simulink model "SimForces2022a"  (R2022a)
settings: Solver=daessc  StartTime=0.0  StopTime=10  FixedStep=0.001  RelTol=1e-4
values from neighbouring files (symbols this model uses):
  Bc1_V = [0;0;0;0;0;0]    [initializeSimulationGP.m]
  D22F = [0;0;0;0;0;0]    [initializeSimulationGP.m]
  filtDV = init2ndOrderLowPassFilter(35*2*pi,1,controller.dT)    [initializeLowPassFilters.m]
  filtEnc = init2ndOrderLowPassFilter(35*2*pi,1,controller.dT)    [initializeLowPassFilters.m]
undefined symbols (not defined in the file or in its folder): aux, B11_r_B11Tc1, B11_V, B11Ftot, B12_r_B12Tc2, B12_Rot_Tc2, B12_U_Tc2, B12_V, B12Ftot, B31_r_B31B41, B31_V, B31FTot, B32_r_B32B42, B32_Rot_B42, B32_U_B42, B32_V, B32FTot, B41_r_B41Tc1, B41_V, B41FTot, B42_r_B42Tc2, B42_Rot_Tc2, B42_U_Tc2, B42_V, B42FTot, B52_r_B52P32, B52_Rot_P32, B52_U_P32, B52_V, B52Ftot, Bc1_r_Bc1B11, Bc1_r_Bc1B31, Bc1FTot, Bc2_r_Bc2B12, Bc2_r_Bc2B32, Bc2_Rot_B12, Bc2_Rot_B32, Bc2_U_B12, Bc2_U_B32, Bc2_V, Bc2Tot, controller, cyl1, cyl2, D22_V, dq1, dq11, dq12, dq2, dq21, dq22, dx1, dx2, dxt2, fc1, fc1r, fc2, fc2r, fct2, fct2r ... (+61)
libraries: sm_lib x32, nesl_utility x20
(part 7 of 7)

== matlab function SimForces2022a/sbVDCController/sbFormAnalyticQuantities/sbRevoluteSegment1/sbGeomPropRS1/sbLiftPistonVelocity/liftPistonVelocity ==
  data: dq1 input; x1 input; q1 input; dx1 output; geom parameter; cyl1 parameter
function dx1 = liftPistonVelocity(dq1, x1, q1, geom, cyl1)

    % Calculates lift piston velocity per the paper equation (21).
    dx1 = -(geom.L1*geom.L11*sin(q1))/(x1+cyl1.x0)*dq1;

end

== matlab function SimForces2022a/sbVDCController/sbFormAnalyticQuantities/sbRevoluteSegment1/sbGeomPropRS1/sbq11AngleVelocity/q11AngleRate ==
  data: x1 input; q11 input; dx1 input; dq11 output; geom parameter; cyl1 parameter
function dq11 = q11AngleRate(x1, q11, dx1, geom, cyl1)
    
    % Calculates q11 angle rate per the paper equation (22).
    dq11 = -((x1+cyl1.x0)-geom.L1*cos(q11))/((x1+cyl1.x0)*geom.L1*sin(q11))*dx1;

end

== matlab function SimForces2022a/sbVDCController/sbFormAnalyticQuantities/sbRevoluteSegment1/sbGeomPropRS1/sbq12AngleRate/q12AngleRate ==
  data: x1 input; q12 input; dx1 input; dq12 output; geom parameter; cyl1 parameter
function dq12 = q12AngleRate(x1, q12, dx1, geom, cyl1)

    % Calculates q12 angle rate per the paper equation (23). 
    dq12 = -((x1+cyl1.x0)-geom.L11*cos(q12))/((x1+cyl1.x0)*geom.L11*sin(q12))*dx1;

end

== matlab function SimForces2022a/sbVDCController/sbFormAnalyticQuantities/sbRevoluteSegment1/sbPosVecsRS1/B31_r_B31B41 ==
  data: x1 input; B31_r_B31B41 output; posVec parameter
function B31_r_B31B41 = B31_r_B31B41(x1, posVec)

    % position vector of {B41} frame at lift piston tip w.r.t. {B31} frame at 
    % lift cylinder connection point [m]
    B31_r_B31B41 = posVec.B31_r_B31B31p + [x1;0;0];

end

== matlab function SimForces2022a/sbVDCController/sbFormAnalyticQuantities/sbRevoluteSegment1/sbGeomPropRS1/sbLiftPistonStroke/liftPistonStroke ==
  data: q1 input; x1 output; geom parameter; cyl1 parameter
function x1 = liftPistonStroke(q1, geom, cyl1)

    % Calculates lift piston stroke per the paper equation (18).
    x1 = sqrt(geom.L1*geom.L1+geom.L11*geom.L11+2*geom.L1*geom.L11*cos(q1))-cyl1.x0;

end

== matlab function SimForces2022a/sbVDCController/sbFormAnalyticQuantities/sbRevoluteSegment1/sbRotMatsRS1/B41_Rot_Tc1 ==
  data: q12 input; B41_Rot_Tc1 output
function B41_Rot_Tc1 = B41_Rot_Tc1(q12)

B41_Rot_Tc1 = [+cos(q12) -sin(q12) 0;...
               +sin(q12) +cos(q12) 0;...
                   0        0      1];

== matlab function SimForces2022a/sbVDCController/sbFormAnalyticQuantities/sbRevoluteSegment1/sbRotMatsRS1/Bc1_Rot_B11 ==
  data: q1 input; Bc1_Rot_B11 output
function Bc1_Rot_B11 = Bc1_Rot_B11(q1)

Bc1_Rot_B11 = [+cos(q1) -sin(q1) 0;...
               +sin(q1) +cos(q1) 0;...
                  0        0     1];

== matlab function SimForces2022a/sbVDCController/sbFormAnalyticQuantities/sbRevoluteSegment1/sbRotMatsRS1/Bc1_Rot_B31 ==
  data: q11 input; Bc1_Rot_B31 output
function Bc1_Rot_B31 = Bc1_Rot_B31(q11)

Bc1_Rot_B31 = [+cos(q11) -sin(q11) 0;...
               +sin(q11) +cos(q11) 0;...
                   0         0     1];

== matlab function SimForces2022a/sbVDCController/sbFormAnalyticQuantities/sbRevoluteSegment1/sbUMatsRS1/B11_U_Tc1 ==
  data: B11_r_B11Tc1 input; B11_U_Tc1 output; B11_Rot_Tc1 input
function B11_U_Tc1 = B11_U_Tc1(B11_r_B11Tc1, B11_Rot_Tc1)

B11_U_Tc1 = [B11_Rot_Tc1,                    zeros(3);...
             dual(B11_r_B11Tc1)*B11_Rot_Tc1, B11_Rot_Tc1];
   
end
   
function dual_r = dual(ArAB)

dual_r = [0,  -ArAB(3), ArAB(2);...
          ArAB(3), 0, -ArAB(1);...
          -ArAB(2), ArAB(1), 0];

end

== matlab function SimForces2022a/sbVDCController/sbFormAnalyticQuantities/sbRevoluteSegment1/sbUMatsRS1/B31_U_B41 ==
  data: B31_r_B31B41 input; B31_U_B41 output; B31_Rot_B41 input
function B31_U_B41 = B31_U_B41(B31_r_B31B41, B31_Rot_B41)

B31_U_B41 = [B31_Rot_B41,                    zeros(3);...
             dual(B31_r_B31B41)*B31_Rot_B41, B31_Rot_B41];
   
end
   
function dual_r = dual(ArAB)

dual_r = [0,  -ArAB(3), ArAB(2);...
          ArAB(3), 0, -ArAB(1);...
          -ArAB(2), ArAB(1), 0];

end

== matlab function SimForces2022a/sbVDCController/sbFormAnalyticQuantities/sbRevoluteSegment1/sbUMatsRS1/B41_U_Tc1 ==
  data: B41_r_B41Tc1 input; B41_U_Tc1 output; B41_Rot_Tc1 input
function B41_U_Tc1 = B41_U_Tc1(B41_r_B41Tc1, B41_Rot_Tc1)

B41_U_Tc1 = [B41_Rot_Tc1,                    zeros(3);...
             dual(B41_r_B41Tc1)*B41_Rot_Tc1, B41_Rot_Tc1];
   
end
   
function dual_r = dual(ArAB)

dual_r = [0,  -ArAB(3), ArAB(2);...
          ArAB(3), 0, -ArAB(1);...
          -ArAB(2), ArAB(1), 0];

end

== matlab function SimForces2022a/sbVDCController/sbFormAnalyticQuantities/sbRevoluteSegment1/sbUMatsRS1/Bc1_U_B11 ==
  data: Bc1_r_Bc1B11 input; Bc1_U_B11 output; Bc1_Rot_B11 input
function Bc1_U_B11 = Bc1_U_B11(Bc1_r_Bc1B11, Bc1_Rot_B11)

Bc1_U_B11 = [Bc1_Rot_B11,                    zeros(3);...
             dual(Bc1_r_Bc1B11)*Bc1_Rot_B11, Bc1_Rot_B11];
   
end
   
function dual_r = dual(ArAB)

dual_r = [0,  -ArAB(3), ArAB(2);...
          ArAB(3), 0, -ArAB(1);...
          -ArAB(2), ArAB(1), 0];

end

== matlab function SimForces2022a/sbVDCController/sbFormAnalyticQuantities/sbRevoluteSegment1/sbUMatsRS1/Bc1_U_B31 ==
  data: Bc1_r_Bc1B31 input; Bc1_U_B31 output; Bc1_Rot_B31 input
function Bc1_U_B31 = Bc1_U_B31(Bc1_r_Bc1B31, Bc1_Rot_B31)

Bc1_U_B31 = [Bc1_Rot_B31,                    zeros(3);...
             dual(Bc1_r_Bc1B31)*Bc1_Rot_B31, Bc1_Rot_B31];
   
end
   
function dual_r = dual(ArAB)

dual_r = [0,  -ArAB(3), ArAB(2);...
          ArAB(3), 0, -ArAB(1);...
          -ArAB(2), ArAB(1), 0];

end

== matlab function SimForces2022a/sbVDCController/sbFormAnalyticQuantities/sbRevoluteSegment1/sbUMatsRS1/Tc1_U_Bc2 ==
  data: Tc1_r_Tc1Bc2 input; Tc1_U_Bc2 output; Tc1_Rot_Bc2 input
function Tc1_U_Bc2 = Tc1_U_Bc2(Tc1_r_Tc1Bc2, Tc1_Rot_Bc2)

Tc1_U_Bc2 = [Tc1_Rot_Bc2,                    zeros(3);...
             dual(Tc1_r_Tc1Bc2)*Tc1_Rot_Bc2, Tc1_Rot_Bc2];
   
end
   
function dual_r = dual(ArAB)

dual_r = [0,  -ArAB(3), ArAB(2);...
          ArAB(3), 0, -ArAB(1);...
          -ArAB(2), ArAB(1), 0];

end

== matlab function SimForces2022a/sbVDCController/sbFormAnalyticQuantities/sbPrismaticSegment2/sbPosVecsPS2/P22_r_P22B52 ==
  data: xt2 input; P22_r_P22B52 output; posVec parameter
function P22_r_P22B52 = P22_r_P22B52(xt2, posVec)

    % position vector of {B41} frame at lift piston tip w.r.t. {B31} frame at 
    % lift cylinder connection point [m]
    P22_r_P22B52 = posVec.P22_r_P22P22p + [xt2; 0; 0];

end

== matlab function SimForces2022a/sbVDCController/sbFormAnalyticQuantities/sbPrismaticSegment2/sbUMatsPS2/B52_U_P32 ==
  data: B52_r_B52B32 input; B52_U_P32 output; B52_Rot_B32 input
function B52_U_P32 = B52_U_P32(B52_r_B52B32, B52_Rot_B32)

B52_U_P32 = [B52_Rot_B32,                    zeros(3);...
             dual(B52_r_B52B32)*B52_Rot_B32, B52_Rot_B32];
   
end
   
function dual_r = dual(ArAB)

dual_r = [0,  -ArAB(3), ArAB(2);...
          ArAB(3), 0, -ArAB(1);...
          -ArAB(2), ArAB(1), 0];

end

== matlab function SimForces2022a/sbVDCController/sbFormAnalyticQuantities/sbPrismaticSegment2/sbUMatsPS2/P22_U_B52 ==
  data: P22_r_P22B52 input; P22_U_B52 output; P22_Rot_B52 input
function P22_U_B52 = P22_U_B52(P22_r_P22B52, P22_Rot_B52)

P22_U_B52 = [P22_Rot_B52,                    zeros(3);...
             dual(P22_r_P22B52)*P22_Rot_B52, P22_Rot_B52];
   
end
   
function dual_r = dual(ArAB)

dual_r = [0,  -ArAB(3), ArAB(2);...
          ArAB(3), 0, -ArAB(1);...
          -ArAB(2), ArAB(1), 0];

end

== matlab function SimForces2022a/sbVDCController/sbFormAnalyticQuantities/sbRevoluteSegment1/sbGeomPropRS1/sbq11AngleValue/q11AngleValue ==
  data: x1 input; q11 output; geom parameter; cyl1 parameter
function q11 = q11AngleValue(x1, geom, cyl1)

    % Calculates q11-angle per the paper equation (19).
    q11 = -acos((geom.L11*geom.L11-(x1+cyl1.x0)*(x1+cyl1.x0)-geom.L1*geom.L1)/(-2*(x1+cyl1.x0)*geom.L1));

end

== matlab function SimForces2022a/sbVDCController/sbFormAnalyticQuantities/sbPrismaticSegment2/sbUMatsPS2/P32_U_D22 ==
  data: P32_r_P32D22 input; P32_U_D22 output; P32_Rot_D22 input
function P32_U_D22 = P32_U_D22(P32_r_P32D22, P32_Rot_D22)

P32_U_D22 = [P32_Rot_D22,                    zeros(3);...
              dual(P32_r_P32D22)*P32_Rot_D22, P32_Rot_D22];
   
end
   
function dual_r = dual(ArAB)

dual_r = [0,  -ArAB(3), ArAB(2);...
          ArAB(3), 0, -ArAB(1);...
          -ArAB(2), ArAB(1), 0];

end

== matlab function SimForces2022a/sbVDCController/sbFormAnalyticQuantities/sbRevoluteSegment2/sbPosVecsRS2/B32_r_B32B42 ==
  data: x2 input; B32_r_B32B42 output; posVec parameter
function B32_r_B32B42 = B32_r_B32B42(x2, posVec)

B32_r_B32B42 = posVec.B32_r_B32B32p + [x2;0;0];

== matlab function SimForces2022a/sbVDCController/sbFormAnalyticQuantities/sbRevoluteSegment2/sbRotMatsRS2/B42_Rot_Tc2 ==
  data: q22 input; B42_Rot_Tc2 output
function B42_Rot_Tc2 = B42_Rot_Tc2(q22)

B42_Rot_Tc2 = [+cos(q22) -sin(q22) 0;...
               +sin(q22) +cos(q22) 0;...
                   0        0      1];

== matlab function SimForces2022a/sbVDCController/sbFormAnalyticQuantities/sbRevoluteSegment2/sbRotMatsRS2/Bc2_Rot_B12 ==
  data: q2 input; Bc2_Rot_B12 output
function Bc2_Rot_B12 = Bc2_Rot_B12(q2)

Bc2_Rot_B12 = [+cos(q2) -sin(q2) 0;...
               +sin(q2) +cos(q2) 0;...
                  0        0     1];

== matlab function SimForces2022a/sbVDCController/sbFormAnalyticQuantities/sbRevoluteSegment2/sbRotMatsRS2/Bc2_Rot_B32 ==
  data: q21 input; Bc2_Rot_B32 output

function Bc2_Rot_B32 = Bc2_Rot_B32(q21)

Bc2_Rot_B32 = [+cos(q21) -sin(q21) 0;...
               +sin(q21) +cos(q21) 0;...
                   0         0     1];

== matlab function SimForces2022a/sbVDCController/sbFormAnalyticQuantities/sbRevoluteSegment2/sbUMatsRS2/B12_U_Tc2 ==
  data: B12_r_B12Tc2 input; B12_U_Tc2 output; B12_Rot_Tc2 input
function B12_U_Tc2 = B12_U_Tc2(B12_r_B12Tc2, B12_Rot_Tc2)

B12_U_Tc2 = [B12_Rot_Tc2,                    zeros(3);...
             dual(B12_r_B12Tc2)*B12_Rot_Tc2, B12_Rot_Tc2];
   
end
   
function dual_r = dual(ArAB)

dual_r = [0,  -ArAB(3), ArAB(2);...
          ArAB(3), 0, -ArAB(1);...
          -ArAB(2), ArAB(1), 0];

end

== matlab function SimForces2022a/sbVDCController/sbFormAnalyticQuantities/sbRevoluteSegment2/sbUMatsRS2/B32_U_B42 ==
  data: B32_r_B32B42 input; B32_U_B42 output; B32_Rot_B42 input
function B32_U_B42 = B32_U_B42(B32_r_B32B42, B32_Rot_B42)

B32_U_B42 = [B32_Rot_B42,                    zeros(3);...
             dual(B32_r_B32B42)*B32_Rot_B42, B32_Rot_B42];
   
end
   
function dual_r = dual(ArAB)

dual_r = [0,  -ArAB(3), ArAB(2);...
          ArAB(3), 0, -ArAB(1);...
          -ArAB(2), ArAB(1), 0];

end

== matlab function SimForces2022a/sbVDCController/sbFormAnalyticQuantities/sbRevoluteSegment2/sbUMatsRS2/B42_U_Tc2 ==
  data: B42_r_B42Tc2 input; B42_U_Tc2 output; B42_Rot_Tc2 input
function B42_U_Tc2 = B42_U_Tc2(B42_r_B42Tc2, B42_Rot_Tc2)

B42_U_Tc2 = [B42_Rot_Tc2,                    zeros(3);...
             dual(B42_r_B42Tc2)*B42_Rot_Tc2, B42_Rot_Tc2];
   
end
   
function dual_r = dual(ArAB)

dual_r = [0,  -ArAB(3), ArAB(2);...
          ArAB(3), 0, -ArAB(1);...
          -ArAB(2), ArAB(1), 0];

end

== matlab function SimForces2022a/sbVDCController/sbFormAnalyticQuantities/sbRevoluteSegment2/sbUMatsRS2/Bc2_U_B12 ==
  data: Bc2_r_Bc2B12 input; Bc2_U_B12 output; Bc2_Rot_B12 input
function Bc2_U_B12 = Bc2_U_B12(Bc2_r_Bc2B12, Bc2_Rot_B12)

Bc2_U_B12 = [Bc2_Rot_B12,                    zeros(3);...
             dual(Bc2_r_Bc2B12)*Bc2_Rot_B12, Bc2_Rot_B12];
   
end
   
function dual_r = dual(ArAB)

dual_r = [0,  -ArAB(3), ArAB(2);...
          ArAB(3), 0, -ArAB(1);...
          -ArAB(2), ArAB(1), 0];

end

== matlab function SimForces2022a/sbVDCController/sbFormAnalyticQuantities/sbRevoluteSegment2/sbUMatsRS2/Bc2_U_B32 ==
  data: Bc2_r_Bc2B32 input; Bc2_U_B32 output; Bc2_Rot_B32 input
function Bc2_U_B32 = Bc2_U_B32(Bc2_r_Bc2B32, Bc2_Rot_B32)

Bc2_U_B32 = [Bc2_Rot_B32,                    zeros(3);...
             dual(Bc2_r_Bc2B32)*Bc2_Rot_B32, Bc2_Rot_B32];
   
end
   
function dual_r = dual(ArAB)

dual_r = [0,  -ArAB(3), ArAB(2);...
          ArAB(3), 0, -ArAB(1);...
          -ArAB(2), ArAB(1), 0];

end

== matlab function SimForces2022a/sbVDCController/sbFormAnalyticQuantities/sbRevoluteSegment2/sbUMatsRS2/Tc2_U_P22 ==
  data: Tc2_r_Tc2P22 input; Tc2_U_P22 output; Tc2_Rot_P22 input
function Tc2_U_P22 = Tc2_U_P22(Tc2_r_Tc2P22, Tc2_Rot_P22)

Tc2_U_P22 = [Tc2_Rot_P22,                    zeros(3);...
             dual(Tc2_r_Tc2P22)*Tc2_Rot_P22, Tc2_Rot_P22];
   
end
   
function dual_r = dual(ArAB)

dual_r = [0,  -ArAB(3), ArAB(2);...
          ArAB(3), 0, -ArAB(1);...
          -ArAB(2), ArAB(1), 0];

end

== matlab function SimForces2022a/sbVDCController/sbFormTotalRequiredForces/sbTotalRequiredForcesPS2/regressorYP22r ==
  data: P22V input; P22dV input; P22_Rot_W input; gravity parameter; YP22r output
function YP22r  = inertiaRegressor(P22V, P22dV, P22_Rot_W,  gravity)

    % Forms regressor matrix YB42r as described in Appendix A of
    % Zhu, Wen-Hong. Virtual decomposition control: toward hyper degrees
    % of freedom robots. Vol. 60. Springer Science & Business Media, 2010.

    % The code below is not the most apparent 1-to-1 visual mapping to the
    % book equations since it was generated using a symbolic toolbox.

    vxr = P22V(1); vyr = P22V(2); vzr = P22V(3);
    wxr = P22V(4); wyr = P22V(5); wzr = P22V(6);
    
    axr = P22dV(1); ayr = P22dV(2); azr = P22dV(3);
    dwxr = P22dV(4); dwyr = P22dV(5); dwzr = P22dV(6);
    
    wx = P22V(4); wy = P22V(5); wz = P22V(6);
    
    P22g = P22_Rot_W*gravity.Wg;
    
    gx = P22g(1); gy = P22g(2); gz = P22g(3);
    
    Y11 = (-vyr * wz + vzr * wy + axr + gx);
    t5 = (wy * wyr);
    t6 = (wz * wzr);
    Y12 = -t5 - t6;
    t7 = (wxr * wy);
    Y13 = (t7 - dwzr);
    t8 = (wxr * wz);
    Y14  = (t8 + dwyr);
    Y15 = 0;
    Y16 = 0;
    Y17 = 0;
    Y18  = 0;
    Y19 = 0;
    Y110 = 0;
    Y111 = 0;
    Y112 = 0;
    Y113 = 0;
    Y21 = vxr * wz - vzr * wx + ayr + gy;
    t11 = wx * wyr;
    Y22 = t11 + dwzr;
    t12 = wx * wxr;
    Y23 = -t12 - t6;
    t13 = wyr * wz;
    Y24 = t13 - dwxr;
    Y25 = 0;
    Y26 = 0;
    Y27 = 0;
    Y28 = 0;
    Y29 = 0;
    Y210 = 0;
    Y211 = 0;
    Y212 = 0;
    Y213 = 0;
    Y31 = -vxr * wy + vyr * wx + azr + gz;
    t16 = wx * wzr;
    Y32 = t16 - dwyr;
    t17 = wy * wzr;
    Y33 = t17 + dwxr;
    Y34 = -t12 - t5;
    Y35 = 0;
    Y36 = 0;
    Y37 = 0;
    Y38 = 0;
    Y39 = 0;
    Y310 = 0;
    Y311 = 0;
    Y312 = 0;
    Y313 = 0;
    Y41 = 0;
    Y42 = 0;
    Y43 = Y31;
    Y44 = -Y21;
    Y45 = 0;
    Y46 = Y33;
    Y47 = -Y24;
    Y48 = Y32;
    Y49 = -Y22;
    Y410 = -t5 + t6;
    Y411 = t17 - t13 + dwxr;
    Y412 = -t13;
    Y413 = t17;
    Y51 = 0;
    Y52 = -Y43;
    Y53 = 0;
    Y54 = Y11;
    Y55 = -Y48;
    Y56 = 0;
    Y57 = Y14;
    Y58 = -Y46;
    Y59 = t12 - t6;
    Y510 = Y13;
    Y511 = t8;
    Y512 = -t16 + Y511 + dwyr;
    Y513 = -t16;
    Y61 = 0;
    Y62 = Y21;
    Y63 = -Y54;
    Y64 = 0;
    Y65 = Y22;
    Y66 = -Y510;
    Y67 = 0;
    Y68 = -t12 + t5;
    Y69 = Y24;
    Y610 = -Y57;
    Y611 = -t7;
    Y612 = t11;
    Y613 = Y612 + Y611 + dwzr;
    
    
    YP22r = [Y11 Y12 Y13 Y14 Y15 Y16 Y17 Y18 Y19 Y110 Y111 Y112 Y113;...
             Y21 Y22 Y23 Y24 Y25 Y26 Y27 Y28 Y29 Y210 Y211 Y212 Y213;...
             Y31 Y32 Y33 Y34 Y35 Y36 Y37 Y38 Y39 Y310 Y311 Y312 Y313;...
             Y41 Y42 Y43 Y44 Y45 Y46 Y47 Y48 Y49 Y410 Y411 Y412 Y413;...
             Y51 Y52 Y53 Y54 Y55 Y56 Y57 Y58 Y59 Y510 Y511 Y512 Y513;...
             Y61 Y62 Y63 Y64 Y65 Y66 Y67 Y68 Y69 Y610 Y611 Y612 Y613];

end

== matlab function SimForces2022a/sbVDCController/sbAuxiliaryJointAngles/q1Angle ==
  data: theta1Filt input; q1 output; geom parameter
function q1 = q1Angle(theta1Filt, geom)

    % Calculates q1 angle value from the encoder- (or other by means-)
    % obtained angle theta1. 
    q1 = -pi/2 - geom.beta1 - geom.beta2 + theta1Filt;

end

== matlab function SimForces2022a/sbVDCController/sbFormTotalRequiredForces/sbTotalRequiredForcesPS2/regressorYP32r ==
  data: P32V input; P32dV input; P32_Rot_W input; gravity parameter; YP32r output
function YP32r  = inertiaRegressor(P32V, P32dV, P32_Rot_W,  gravity)
    
    % Forms regressor matrix YB42r as described in Appendix A of
    % Zhu, Wen-Hong. Virtual decomposition control: toward hyper degrees
    % of freedom robots. Vol. 60. Springer Science & Business Media, 2010.

    % The code below is not the most apparent 1-to-1 visual mapping to the
    % book equations since it was generated using a symbolic toolbox.

    vxr = P32V(1); vyr = P32V(2); vzr = P32V(3);
    wxr = P32V(4); wyr = P32V(5); wzr = P32V(6);
    
    axr = P32dV(1); ayr = P32dV(2); azr = P32dV(3);
    dwxr = P32dV(4); dwyr = P32dV(5); dwzr = P32dV(6);
    
    wx = P32V(4); wy = P32V(5); wz = P32V(6);
    
    P32g = P32_Rot_W*gravity.Wg;
    
    gx = P32g(1); gy = P32g(2); gz = P32g(3);
    
    Y11 = (-vyr * wz + vzr * wy + axr + gx);
    t5 = (wy * wyr);
    t6 = (wz * wzr);
    Y12 = -t5 - t6;
    t7 = (wxr * wy);
    Y13 = (t7 - dwzr);
    t8 = (wxr * wz);
    Y14  = (t8 + dwyr);
    Y15 = 0;
    Y16 = 0;
    Y17 = 0;
    Y18  = 0;
    Y19 = 0;
    Y110 = 0;
    Y111 = 0;
    Y112 = 0;
    Y113 = 0;
    Y21 = vxr * wz - vzr * wx + ayr + gy;
    t11 = wx * wyr;
    Y22 = t11 + dwzr;
    t12 = wx * wxr;
    Y23 = -t12 - t6;
    t13 = wyr * wz;
    Y24 = t13 - dwxr;
    Y25 = 0;
    Y26 = 0;
    Y27 = 0;
    Y28 = 0;
    Y29 = 0;
    Y210 = 0;
    Y211 = 0;
    Y212 = 0;
    Y213 = 0;
    Y31 = -vxr * wy + vyr * wx + azr + gz;
    t16 = wx * wzr;
    Y32 = t16 - dwyr;
    t17 = wy * wzr;
    Y33 = t17 + dwxr;
    Y34 = -t12 - t5;
    Y35 = 0;
    Y36 = 0;
    Y37 = 0;
    Y38 = 0;
    Y39 = 0;
    Y310 = 0;
    Y311 = 0;
    Y312 = 0;
    Y313 = 0;
    Y41 = 0;
    Y42 = 0;
    Y43 = Y31;
    Y44 = -Y21;
    Y45 = 0;
    Y46 = Y33;
    Y47 = -Y24;
    Y48 = Y32;
    Y49 = -Y22;
    Y410 = -t5 + t6;
    Y411 = t17 - t13 + dwxr;
    Y412 = -t13;
    Y413 = t17;
    Y51 = 0;
    Y52 = -Y43;
    Y53 = 0;
    Y54 = Y11;
    Y55 = -Y48;
    Y56 = 0;
    Y57 = Y14;
    Y58 = -Y46;
    Y59 = t12 - t6;
    Y510 = Y13;
    Y511 = t8;
    Y512 = -t16 + Y511 + dwyr;
    Y513 = -t16;
    Y61 = 0;
    Y62 = Y21;
    Y63 = -Y54;
    Y64 = 0;
    Y65 = Y22;
    Y66 = -Y510;
    Y67 = 0;
    Y68 = -t12 + t5;
    Y69 = Y24;
    Y610 = -Y57;
    Y611 = -t7;
    Y612 = t11;
    Y613 = Y612 + Y611 + dwzr;
    
    
    YP32r = [Y11 Y12 Y13 Y14 Y15 Y16 Y17 Y18 Y19 Y110 Y111 Y112 Y113;...
         Y21 Y22 Y23 Y24 Y25 Y26 Y27 Y28 Y29 Y210 Y211 Y212 Y213;...
         Y31 Y32 Y33 Y34 Y35 Y36 Y37 Y38 Y39 Y310 Y311 Y312 Y313;...
         Y41 Y42 Y43 Y44 Y45 Y46 Y47 Y48 Y49 Y410 Y411 Y412 Y413;...
         Y51 Y52 Y53 Y54 Y55 Y56 Y57 Y58 Y59 Y510 Y511 Y512 Y513;...
         Y61 Y62 Y63 Y64 Y65 Y66 Y67 Y68 Y69 Y610 Y611 Y612 Y613];

end

== matlab function SimForces2022a/sbVDCController/sbFormTotalRequiredForces/sbTotalRequiredForcesRS2/regressorYB12r ==
  data: B12V input; B12dV input; B12_Rot_W input; gravity parameter; YB12r output
function YB12r  = inertiaRegressor(B12V, B12dV, B12_Rot_W,  gravity)

    % Forms regressor matrix YB12r as described in Appendix A of
    % Zhu, Wen-Hong. Virtual decomposition control: toward hyper degrees
    % of freedom robots. Vol. 60. Springer Science & Business Media, 2010.

    % The code below is not the most apparent 1-to-1 visual mapping to the
    % book equations since it was generated using a symbolic toolbox.

    vxr = B12V(1); vyr = B12V(2); vzr = B12V(3);
    wxr = B12V(4); wyr = B12V(5); wzr = B12V(6);
    
    axr = B12dV(1); ayr = B12dV(2); azr = B12dV(3);
    dwxr = B12dV(4); dwyr = B12dV(5); dwzr = B12dV(6);
    
    wx = B12V(4); wy = B12V(5); wz = B12V(6);
    
    B12g = B12_Rot_W*gravity.Wg;
    
    gx = B12g(1); gy = B12g(2); gz = B12g(3);
    
    Y11 = (-vyr * wz + vzr * wy + axr + gx);
    t5 = (wy * wyr);
    t6 = (wz * wzr);
    Y12 = -t5 - t6;
    t7 = (wxr * wy);
    Y13 = (t7 - dwzr);
    t8 = (wxr * wz);
    Y14  = (t8 + dwyr);
    Y15 = 0;
    Y16 = 0;
    Y17 = 0;
    Y18  = 0;
    Y19 = 0;
    Y110 = 0;
    Y111 = 0;
    Y112 = 0;
    Y113 = 0;
    Y21 = vxr * wz - vzr * wx + ayr + gy;
    t11 = wx * wyr;
    Y22 = t11 + dwzr;
    t12 = wx * wxr;
    Y23 = -t12 - t6;
    t13 = wyr * wz;
    Y24 = t13 - dwxr;
    Y25 = 0;
    Y26 = 0;
    Y27 = 0;
    Y28 = 0;
    Y29 = 0;
    Y210 = 0;
    Y211 = 0;
    Y212 = 0;
    Y213 = 0;
    Y31 = -vxr * wy + vyr * wx + azr + gz;
    t16 = wx * wzr;
    Y32 = t16 - dwyr;
    t17 = wy * wzr;
    Y33 = t17 + dwxr;
    Y34 = -t12 - t5;
    Y35 = 0;
    Y36 = 0;
    Y37 = 0;
    Y38 = 0;
    Y39 = 0;
    Y310 = 0;
    Y311 = 0;
    Y312 = 0;
    Y313 = 0;
    Y41 = 0;
    Y42 = 0;
    Y43 = Y31;
    Y44 = -Y21;
    Y45 = 0;
    Y46 = Y33;
    Y47 = -Y24;
    Y48 = Y32;
    Y49 = -Y22;
    Y410 = -t5 + t6;
    Y411 = t17 - t13 + dwxr;
    Y412 = -t13;
    Y413 = t17;
    Y51 = 0;
    Y52 = -Y43;
    Y53 = 0;
    Y54 = Y11;
    Y55 = -Y48;
    Y56 = 0;
    Y57 = Y14;
    Y58 = -Y46;
    Y59 = t12 - t6;
    Y510 = Y13;
    Y511 = t8;
    Y512 = -t16 + Y511 + dwyr;
    Y513 = -t16;
    Y61 = 0;
    Y62 = Y21;
    Y63 = -Y54;
    Y64 = 0;
    Y65 = Y22;
    Y66 = -Y510;
    Y67 = 0;
    Y68 = -t12 + t5;
    Y69 = Y24;
    Y610 = -Y57;
    Y611 = -t7;
    Y612 = t11;
    Y613 = Y612 + Y611 + dwzr;
    
    
    YB12r = [Y11 Y12 Y13 Y14 Y15 Y16 Y17 Y18 Y19 Y110 Y111 Y112 Y113;...
    	     Y21 Y22 Y23 Y24 Y25 Y26 Y27 Y28 Y29 Y210 Y211 Y212 Y213;...
             Y31 Y32 Y33 Y34 Y35 Y36 Y37 Y38 Y39 Y310 Y311 Y312 Y313;...
             Y41 Y42 Y43 Y44 Y45 Y46 Y47 Y48 Y49 Y410 Y411 Y412 Y413;...
             Y51 Y52 Y53 Y54 Y55 Y56 Y57 Y58 Y59 Y510 Y511 Y512 Y513;...
             Y61 Y62 Y63 Y64 Y65 Y66 Y67 Y68 Y69 Y610 Y611 Y612 Y613];

end

== matlab function SimForces2022a/sbVDCController/sbFormTotalRequiredForces/sbTotalRequiredForcesRS2/regressorYB32r ==
  data: B32V input; B32dV input; B32_Rot_W input; gravity parameter; YB32r output
function YB32r  = YB32r(B32V, B32dV, B32_Rot_W,  gravity)

    % Forms regressor matrix YB32r as described in Appendix A of
    % Zhu, Wen-Hong. Virtual decomposition control: toward hyper degrees
    % of freedom robots. Vol. 60. Springer Science & Business Media, 2010.

    % The code below is not the most apparent 1-to-1 visual mapping to the
    % book equations since it was generated using a symbolic toolbox.

    vxr = B32V(1); vyr = B32V(2); vzr = B32V(3);
    wxr = B32V(4); wyr = B32V(5); wzr = B32V(6);
    
    axr = B32dV(1); ayr = B32dV(2); azr = B32dV(3);
    dwxr = B32dV(4); dwyr = B32dV(5); dwzr = B32dV(6);
    
    wx = B32V(4); wy = B32V(5); wz = B32V(6);
    
    B32g = B32_Rot_W*gravity.Wg;
    
    gx = B32g(1); gy = B32g(2); gz = B32g(3);
    
    Y11 = (-vyr * wz + vzr * wy + axr + gx);
    t5 = (wy * wyr);
    t6 = (wz * wzr);
    Y12 = -t5 - t6;
    t7 = (wxr * wy);
    Y13 = (t7 - dwzr);
    t8 = (wxr * wz);
    Y14  = (t8 + dwyr);
    Y15 = 0;
    Y16 = 0;
    Y17 = 0;
    Y18  = 0;
    Y19 = 0;
    Y110 = 0;
    Y111 = 0;
    Y112 = 0;
    Y113 = 0;
    Y21 = vxr * wz - vzr * wx + ayr + gy;
    t11 = wx * wyr;
    Y22 = t11 + dwzr;
    t12 = wx * wxr;
    Y23 = -t12 - t6;
    t13 = wyr * wz;
    Y24 = t13 - dwxr;
    Y25 = 0;
    Y26 = 0;
    Y27 = 0;
    Y28 = 0;
    Y29 = 0;
    Y210 = 0;
    Y211 = 0;
    Y212 = 0;
    Y213 = 0;
    Y31 = -vxr * wy + vyr * wx + azr + gz;
    t16 = wx * wzr;
    Y32 = t16 - dwyr;
    t17 = wy * wzr;
    Y33 = t17 + dwxr;
    Y34 = -t12 - t5;
    Y35 = 0;
    Y36 = 0;
    Y37 = 0;
    Y38 = 0;
    Y39 = 0;
    Y310 = 0;
    Y311 = 0;
    Y312 = 0;
    Y313 = 0;
    Y41 = 0;
    Y42 = 0;
    Y43 = Y31;
    Y44 = -Y21;
    Y45 = 0;
    Y46 = Y33;
    Y47 = -Y24;
    Y48 = Y32;
    Y49 = -Y22;
    Y410 = -t5 + t6;
    Y411 = t17 - t13 + dwxr;
    Y412 = -t13;
    Y413 = t17;
    Y51 = 0;
    Y52 = -Y43;
    Y53 = 0;
    Y54 = Y11;
    Y55 = -Y48;
    Y56 = 0;
    Y57 = Y14;
    Y58 = -Y46;
    Y59 = t12 - t6;
    Y510 = Y13;
    Y511 = t8;
    Y512 = -t16 + Y511 + dwyr;
    Y513 = -t16;
    Y61 = 0;
    Y62 = Y21;
    Y63 = -Y54;
    Y64 = 0;
    Y65 = Y22;
    Y66 = -Y510;
    Y67 = 0;
    Y68 = -t12 + t5;
    Y69 = Y24;
    Y610 = -Y57;
    Y611 = -t7;
    Y612 = t11;
    Y613 = Y612 + Y611 + dwzr;
    
    
    YB32r = [Y11 Y12 Y13 Y14 Y15 Y16 Y17 Y18 Y19 Y110 Y111 Y112 Y113;...
             Y21 Y22 Y23 Y24 Y25 Y26 Y27 Y28 Y29 Y210 Y211 Y212 Y213;...
             Y31 Y32 Y33 Y34 Y35 Y36 Y37 Y38 Y39 Y310 Y311 Y312 Y313;...
             Y41 Y42 Y43 Y44 Y45 Y46 Y47 Y48 Y49 Y410 Y411 Y412 Y413;...
             Y51 Y52 Y53 Y54 Y55 Y56 Y57 Y58 Y59 Y510 Y511 Y512 Y513;...
             Y61 Y62 Y63 Y64 Y65 Y66 Y67 Y68 Y69 Y610 Y611 Y612 Y613];

end

== matlab function SimForces2022a/sbVDCController/sbFormTotalRequiredForces/sbTotalRequiredForcesRS2/regressorYB42r ==
  data: B42V input; B42dV input; B42_Rot_W input; gravity parameter; YB42r output
function YB42r  = inertiaRegressor(B42V, B42dV, B42_Rot_W,  gravity)

    % Forms regressor matrix YB42r as described in Appendix A of
    % Zhu, Wen-Hong. Virtual decomposition control: toward hyper degrees
    % of freedom robots. Vol. 60. Springer Science & Business Media, 2010.

    % The code below is not the most apparent 1-to-1 visual mapping to the
    % book equations since it was generated using a symbolic toolbox.

    vxr = B42V(1); vyr = B42V(2); vzr = B42V(3);
    wxr = B42V(4); wyr = B42V(5); wzr = B42V(6);
    
    axr = B42dV(1); ayr = B42dV(2); azr = B42dV(3);
    dwxr = B42dV(4); dwyr = B42dV(5); dwzr = B42dV(6);
    
    wx = B42V(4); wy = B42V(5); wz = B42V(6);
    
    B42g = B42_Rot_W*gravity.Wg;
    
    gx = B42g(1); gy = B42g(2); gz = B42g(3);
    
    Y11 = (-vyr * wz + vzr * wy + axr + gx);
    t5 = (wy * wyr);
    t6 = (wz * wzr);
    Y12 = -t5 - t6;
    t7 = (wxr * wy);
    Y13 = (t7 - dwzr);
    t8 = (wxr * wz);
    Y14  = (t8 + dwyr);
    Y15 = 0;
    Y16 = 0;
    Y17 = 0;
    Y18  = 0;
    Y19 = 0;
    Y110 = 0;
    Y111 = 0;
    Y112 = 0;
    Y113 = 0;
    Y21 = vxr * wz - vzr * wx + ayr + gy;
    t11 = wx * wyr;
    Y22 = t11 + dwzr;
    t12 = wx * wxr;
    Y23 = -t12 - t6;
    t13 = wyr * wz;
    Y24 = t13 - dwxr;
    Y25 = 0;
    Y26 = 0;
    Y27 = 0;
    Y28 = 0;
    Y29 = 0;
    Y210 = 0;
    Y211 = 0;
    Y212 = 0;
    Y213 = 0;
    Y31 = -vxr * wy + vyr * wx + azr + gz;
    t16 = wx * wzr;
    Y32 = t16 - dwyr;
    t17 = wy * wzr;
    Y33 = t17 + dwxr;
    Y34 = -t12 - t5;
    Y35 = 0;
    Y36 = 0;
    Y37 = 0;
    Y38 = 0;
    Y39 = 0;
    Y310 = 0;
    Y311 = 0;
    Y312 = 0;
    Y313 = 0;
    Y41 = 0;
    Y42 = 0;
    Y43 = Y31;
    Y44 = -Y21;
    Y45 = 0;
    Y46 = Y33;
    Y47 = -Y24;
    Y48 = Y32;
    Y49 = -Y22;
    Y410 = -t5 + t6;
    Y411 = t17 - t13 + dwxr;
    Y412 = -t13;
    Y413 = t17;
    Y51 = 0;
    Y52 = -Y43;
    Y53 = 0;
    Y54 = Y11;
    Y55 = -Y48;
    Y56 = 0;
    Y57 = Y14;
    Y58 = -Y46;
    Y59 = t12 - t6;
    Y510 = Y13;
    Y511 = t8;
    Y512 = -t16 + Y511 + dwyr;
    Y513 = -t16;
    Y61 = 0;
    Y62 = Y21;
    Y63 = -Y54;
    Y64 = 0;
    Y65 = Y22;
    Y66 = -Y510;
    Y67 = 0;
    Y68 = -t12 + t5;
    Y69 = Y24;
    Y610 = -Y57;
    Y611 = -t7;
    Y612 = t11;
    Y613 = Y612 + Y611 + dwzr;
    
    
    YB42r = [Y11 Y12 Y13 Y14 Y15 Y16 Y17 Y18 Y19 Y110 Y111 Y112 Y113;...
             Y21 Y22 Y23 Y24 Y25 Y26 Y27 Y28 Y29 Y210 Y211 Y212 Y213;...
             Y31 Y32 Y33 Y34 Y35 Y36 Y37 Y38 Y39 Y310 Y311 Y312 Y313;...
             Y41 Y42 Y43 Y44 Y45 Y46 Y47 Y48 Y49 Y410 Y411 Y412 Y413;...
             Y51 Y52 Y53 Y54 Y55 Y56 Y57 Y58 Y59 Y510 Y511 Y512 Y513;...
             Y61 Y62 Y63 Y64 Y65 Y66 Y67 Y68 Y69 Y610 Y611 Y612 Y613];

end

== matlab function SimForces2022a/sbVDCController/sbFormTotalRequiredForces/sbTotalRequiredForcesRS2/regressorYBc2r ==
  data: Bc2V input; Bc2dV input; Bc2_Rot_W input; gravity parameter; YBc2r output
function YBc2r  = inertiaRegressor(Bc2V, Bc2dV, Bc2_Rot_W,  gravity)

    % Forms regressor matrix YBc2r as described in Appendix A of
    % Zhu, Wen-Hong. Virtual decomposition control: toward hyper degrees
    % of freedom robots. Vol. 60. Springer Science & Business Media, 2010.

    % The code below is not the most apparent 1-to-1 visual mapping to the
    % book equations since it was generated using a symbolic toolbox.

    vxr = Bc2V(1); vyr = Bc2V(2); vzr = Bc2V(3);
    wxr = Bc2V(4); wyr = Bc2V(5); wzr = Bc2V(6);
    
    axr = Bc2dV(1); ayr = Bc2dV(2); azr = Bc2dV(3);
    dwxr = Bc2dV(4); dwyr = Bc2dV(5); dwzr = Bc2dV(6);
    
    wx = Bc2V(4); wy = Bc2V(5); wz = Bc2V(6);
    
    Bc2g = Bc2_Rot_W*gravity.Wg;
    
    gx = Bc2g(1); gy = Bc2g(2); gz = Bc2g(3);
    
    Y11 = (-vyr * wz + vzr * wy + axr + gx);
    t5 = (wy * wyr);
    t6 = (wz * wzr);
    Y12 = -t5 - t6;
    t7 = (wxr * wy);
    Y13 = (t7 - dwzr);
    t8 = (wxr * wz);
    Y14  = (t8 + dwyr);
    Y15 = 0;
    Y16 = 0;
    Y17 = 0;
    Y18  = 0;
    Y19 = 0;
    Y110 = 0;
    Y111 = 0;
    Y112 = 0;
    Y113 = 0;
    Y21 = vxr * wz - vzr * wx + ayr + gy;
    t11 = wx * wyr;
    Y22 = t11 + dwzr;
    t12 = wx * wxr;
    Y23 = -t12 - t6;
    t13 = wyr * wz;
    Y24 = t13 - dwxr;
    Y25 = 0;
    Y26 = 0;
    Y27 = 0;
    Y28 = 0;
    Y29 = 0;
    Y210 = 0;
    Y211 = 0;
    Y212 = 0;
    Y213 = 0;
    Y31 = -vxr * wy + vyr * wx + azr + gz;
    t16 = wx * wzr;
    Y32 = t16 - dwyr;
    t17 = wy * wzr;
    Y33 = t17 + dwxr;
    Y34 = -t12 - t5;
    Y35 = 0;
    Y36 = 0;
    Y37 = 0;
    Y38 = 0;
    Y39 = 0;
    Y310 = 0;
    Y311 = 0;
    Y312 = 0;
    Y313 = 0;
    Y41 = 0;
    Y42 = 0;
    Y43 = Y31;
    Y44 = -Y21;
    Y45 = 0;
    Y46 = Y33;
    Y47 = -Y24;
    Y48 = Y32;
    Y49 = -Y22;
    Y410 = -t5 + t6;
    Y411 = t17 - t13 + dwxr;
    Y412 = -t13;
    Y413 = t17;
    Y51 = 0;
    Y52 = -Y43;
    Y53 = 0;
    Y54 = Y11;
    Y55 = -Y48;
    Y56 = 0;
    Y57 = Y14;
    Y58 = -Y46;
    Y59 = t12 - t6;
    Y510 = Y13;
    Y511 = t8;
    Y512 = -t16 + Y511 + dwyr;
    Y513 = -t16;
    Y61 = 0;
    Y62 = Y21;
    Y63 = -Y54;
    Y64 = 0;
    Y65 = Y22;
    Y66 = -Y510;
    Y67 = 0;
    Y68 = -t12 + t5;
    Y69 = Y24;
    Y610 = -Y57;
    Y611 = -t7;
    Y612 = t11;
    Y613 = Y612 + Y611 + dwzr;
    
    
    YBc2r = [Y11 Y12 Y13 Y14 Y15 Y16 Y17 Y18 Y19 Y110 Y111 Y112 Y113;...
             Y21 Y22 Y23 Y24 Y25 Y26 Y27 Y28 Y29 Y210 Y211 Y212 Y213;...
             Y31 Y32 Y33 Y34 Y35 Y36 Y37 Y38 Y39 Y310 Y311 Y312 Y313;...
             Y41 Y42 Y43 Y44 Y45 Y46 Y47 Y48 Y49 Y410 Y411 Y412 Y413;...
             Y51 Y52 Y53 Y54 Y55 Y56 Y57 Y58 Y59 Y510 Y511 Y512 Y513;...
             Y61 Y62 Y63 Y64 Y65 Y66 Y67 Y68 Y69 Y610 Y611 Y612 Y613];

end

== matlab function SimForces2022a/sbVDCController/sbFormTotalRequiredForces/sbTotalRequiredForcesRS1/regressorYB11r ==
  data: B11V input; B11dV input; B11_Rot_W input; gravity parameter; YB11r output
function YB11r  = inertiaRegressor(B11V, B11dV, B11_Rot_W,  gravity)

    % Forms regressor matrix YB11r as described in Appendix A of
    % Zhu, Wen-Hong. Virtual decomposition control: toward hyper degrees
    % of freedom robots. Vol. 60. Springer Science & Business Media, 2010.

    % The code below is not the most apparent 1-to-1 visual mapping to the
    % book equations since it was generated using a symbolic toolbox.
    
    vxr = B11V(1); vyr = B11V(2); vzr = B11V(3);
    wxr = B11V(4); wyr = B11V(5); wzr = B11V(6);
    
    axr = B11dV(1); ayr = B11dV(2); azr = B11dV(3);
    dwxr = B11dV(4); dwyr = B11dV(5); dwzr = B11dV(6);
    
    wx = B11V(4); wy = B11V(5); wz = B11V(6);
    
    B11g = B11_Rot_W*gravity.Wg;
    
    gx = B11g(1); gy = B11g(2); gz = B11g(3);
    
    Y11 = (-vyr * wz + vzr * wy + axr + gx);
    t5 = (wy * wyr);
    t6 = (wz * wzr);
    Y12 = -t5 - t6;
    t7 = (wxr * wy);
    Y13 = (t7 - dwzr);
    t8 = (wxr * wz);
    Y14  = (t8 + dwyr);
    Y15 = 0;
    Y16 = 0;
    Y17 = 0;
    Y18  = 0;
    Y19 = 0;
    Y110 = 0;
    Y111 = 0;
    Y112 = 0;
    Y113 = 0;
    Y21 = vxr * wz - vzr * wx + ayr + gy;
    t11 = wx * wyr;
    Y22 = t11 + dwzr;
    t12 = wx * wxr;
    Y23 = -t12 - t6;
    t13 = wyr * wz;
    Y24 = t13 - dwxr;
    Y25 = 0;
    Y26 = 0;
    Y27 = 0;
    Y28 = 0;
    Y29 = 0;
    Y210 = 0;
    Y211 = 0;
    Y212 = 0;
    Y213 = 0;
    Y31 = -vxr * wy + vyr * wx + azr + gz;
    t16 = wx * wzr;
    Y32 = t16 - dwyr;
    t17 = wy * wzr;
    Y33 = t17 + dwxr;
    Y34 = -t12 - t5;
    Y35 = 0;
    Y36 = 0;
    Y37 = 0;
    Y38 = 0;
    Y39 = 0;
    Y310 = 0;
    Y311 = 0;
    Y312 = 0;
    Y313 = 0;
    Y41 = 0;
    Y42 = 0;
    Y43 = Y31;
    Y44 = -Y21;
    Y45 = 0;
    Y46 = Y33;
    Y47 = -Y24;
    Y48 = Y32;
    Y49 = -Y22;
    Y410 = -t5 + t6;
    Y411 = t17 - t13 + dwxr;
    Y412 = -t13;
    Y413 = t17;
    Y51 = 0;
    Y52 = -Y43;
    Y53 = 0;
    Y54 = Y11;
    Y55 = -Y48;
    Y56 = 0;
    Y57 = Y14;
    Y58 = -Y46;
    Y59 = t12 - t6;
    Y510 = Y13;
    Y511 = t8;
    Y512 = -t16 + Y511 + dwyr;
    Y513 = -t16;
    Y61 = 0;
    Y62 = Y21;
    Y63 = -Y54;
    Y64 = 0;
    Y65 = Y22;
    Y66 = -Y510;
    Y67 = 0;
    Y68 = -t12 + t5;
    Y69 = Y24;
    Y610 = -Y57;
    Y611 = -t7;
    Y612 = t11;
    Y613 = Y612 + Y611 + dwzr;
    
    
    YB11r = [Y11 Y12 Y13 Y14 Y15 Y16 Y17 Y18 Y19 Y110 Y111 Y112 Y113;...
             Y21 Y22 Y23 Y24 Y25 Y26 Y27 Y28 Y29 Y210 Y211 Y212 Y213;...
             Y31 Y32 Y33 Y34 Y35 Y36 Y37 Y38 Y39 Y310 Y311 Y312 Y313;...
             Y41 Y42 Y43 Y44 Y45 Y46 Y47 Y48 Y49 Y410 Y411 Y412 Y413;...
             Y51 Y52 Y53 Y54 Y55 Y56 Y57 Y58 Y59 Y510 Y511 Y512 Y513;...
             Y61 Y62 Y63 Y64 Y65 Y66 Y67 Y68 Y69 Y610 Y611 Y612 Y613];

end

== matlab function SimForces2022a/sbVDCController/sbFormTotalRequiredForces/sbTotalRequiredForcesRS1/regressorYB31r ==
  data: B31V input; B31dV input; B31_Rot_W input; gravity parameter; YB31r output
function YB31r  = inertiaRegressor(B31V, B31dV, B31_Rot_W,  gravity)

    % Forms regressor matrix YB31r as described in Appendix A of
    % Zhu, Wen-Hong. Virtual decomposition control: toward hyper degrees
    % of freedom robots. Vol. 60. Springer Science & Business Media, 2010.

    % The code below is not the most apparent 1-to-1 visual mapping to the
    % book equations since it was generated using a symbolic toolbox.

    vxr = B31V(1); vyr = B31V(2); vzr = B31V(3);
    wxr = B31V(4); wyr = B31V(5); wzr = B31V(6);
    
    axr = B31dV(1); ayr = B31dV(2); azr = B31dV(3);
    dwxr = B31dV(4); dwyr = B31dV(5); dwzr = B31dV(6); 
    
    wx = B31V(4); wy = B31V(5); wz = B31V(6);
    
    B31g = B31_Rot_W*gravity.Wg;
    
    gx = B31g(1); gy = B31g(2); gz = B31g(3);
    
    Y11 = (-vyr * wz + vzr * wy + axr + gx);
    t5 = (wy * wyr);
    t6 = (wz * wzr);
    Y12 = -t5 - t6;
    t7 = (wxr * wy);
    Y13 = (t7 - dwzr);
    t8 = (wxr * wz);
    Y14  = (t8 + dwyr);
    Y15 = 0;
    Y16 = 0;
    Y17 = 0;
    Y18  = 0;
    Y19 = 0;
    Y110 = 0;
    Y111 = 0;
    Y112 = 0;
    Y113 = 0;
    Y21 = vxr * wz - vzr * wx + ayr + gy;
    t11 = wx * wyr;
    Y22 = t11 + dwzr;
    t12 = wx * wxr;
    Y23 = -t12 - t6;
    t13 = wyr * wz;
    Y24 = t13 - dwxr;
    Y25 = 0;
    Y26 = 0;
    Y27 = 0;
    Y28 = 0;
    Y29 = 0;
    Y210 = 0;
    Y211 = 0;
    Y212 = 0;
    Y213 = 0;
    Y31 = -vxr * wy + vyr * wx + azr + gz;
    t16 = wx * wzr;
    Y32 = t16 - dwyr;
    t17 = wy * wzr;
    Y33 = t17 + dwxr;
    Y34 = -t12 - t5;
    Y35 = 0;
    Y36 = 0;
    Y37 = 0;
    Y38 = 0;
    Y39 = 0;
    Y310 = 0;
    Y311 = 0;
    Y312 = 0;
    Y313 = 0;
    Y41 = 0;
    Y42 = 0;
    Y43 = Y31;
    Y44 = -Y21;
    Y45 = 0;
    Y46 = Y33;
    Y47 = -Y24;
    Y48 = Y32;
    Y49 = -Y22;
    Y410 = -t5 + t6;
    Y411 = t17 - t13 + dwxr;
    Y412 = -t13;
    Y413 = t17;
    Y51 = 0;
    Y52 = -Y43;
    Y53 = 0;
    Y54 = Y11;
    Y55 = -Y48;
    Y56 = 0;
    Y57 = Y14;
    Y58 = -Y46;
    Y59 = t12 - t6;
    Y510 = Y13;
    Y511 = t8;
    Y512 = -t16 + Y511 + dwyr;
    Y513 = -t16;
    Y61 = 0;
    Y62 = Y21;
    Y63 = -Y54;
    Y64 = 0;
    Y65 = Y22;
    Y66 = -Y510;
    Y67 = 0;
    Y68 = -t12 + t5;
    Y69 = Y24;
    Y610 = -Y57;
    Y611 = -t7;
    Y612 = t11;
    Y613 = Y612 + Y611 + dwzr;
    
    
    YB31r = [Y11 Y12 Y13 Y14 Y15 Y16 Y17 Y18 Y19 Y110 Y111 Y112 Y113;...
             Y21 Y22 Y23 Y24 Y25 Y26 Y27 Y28 Y29 Y210 Y211 Y212 Y213;...
             Y31 Y32 Y33 Y34 Y35 Y36 Y37 Y38 Y39 Y310 Y311 Y312 Y313;...
             Y41 Y42 Y43 Y44 Y45 Y46 Y47 Y48 Y49 Y410 Y411 Y412 Y413;...
             Y51 Y52 Y53 Y54 Y55 Y56 Y57 Y58 Y59 Y510 Y511 Y512 Y513;...
             Y61 Y62 Y63 Y64 Y65 Y66 Y67 Y68 Y69 Y610 Y611 Y612 Y613];

end

== matlab function SimForces2022a/sbVDCController/sbFormTotalRequiredForces/sbTotalRequiredForcesRS1/regressorYB41r ==
  data: B41V input; B41dV input; B41_Rot_W input; gravity parameter; YB41r output
function YB41r  = inertiaRegressor(B41V, B41dV, B41_Rot_W,  gravity)

    % Forms regressor matrix YB41r as described in Appendix A of
    % Zhu, Wen-Hong. Virtual decomposition control: toward hyper degrees
    % of freedom robots. Vol. 60. Springer Science & Business Media, 2010.

    % The code below is not the most apparent 1-to-1 visual mapping to the
    % book equations since it was generated using a symbolic toolbox.
    
    vxr = B41V(1); vyr = B41V(2); vzr = B41V(3);
    wxr = B41V(4); wyr = B41V(5); wzr = B41V(6);
    
    axr = B41dV(1); ayr = B41dV(2); azr = B41dV(3);
    dwxr = B41dV(4); dwyr = B41dV(5); dwzr = B41dV(6);
    
    wx = B41V(4); wy = B41V(5); wz = B41V(6);
    
    B41g = B41_Rot_W*gravity.Wg;
    
    gx = B41g(1);
    gy = B41g(2);
    gz = B41g(3);
    
    Y11 = (-vyr * wz + vzr * wy + axr + gx);
    t5 = (wy * wyr);
    t6 = (wz * wzr);
    Y12 = -t5 - t6;
    t7 = (wxr * wy);
    Y13 = (t7 - dwzr);
    t8 = (wxr * wz);
    Y14  = (t8 + dwyr);
    Y15 = 0;
    Y16 = 0;
    Y17 = 0;
    Y18  = 0;
    Y19 = 0;
    Y110 = 0;
    Y111 = 0;
    Y112 = 0;
    Y113 = 0;
    Y21 = vxr * wz - vzr * wx + ayr + gy;
    t11 = wx * wyr;
    Y22 = t11 + dwzr;
    t12 = wx * wxr;
    Y23 = -t12 - t6;
    t13 = wyr * wz;
    Y24 = t13 - dwxr;
    Y25 = 0;
    Y26 = 0;
    Y27 = 0;
    Y28 = 0;
    Y29 = 0;
    Y210 = 0;
    Y211 = 0;
    Y212 = 0;
    Y213 = 0;
    Y31 = -vxr * wy + vyr * wx + azr + gz;
    t16 = wx * wzr;
    Y32 = t16 - dwyr;
    t17 = wy * wzr;
    Y33 = t17 + dwxr;
    Y34 = -t12 - t5;
    Y35 = 0;
    Y36 = 0;
    Y37 = 0;
    Y38 = 0;
    Y39 = 0;
    Y310 = 0;
    Y311 = 0;
    Y312 = 0;
    Y313 = 0;
    Y41 = 0;
    Y42 = 0;
    Y43 = Y31;
    Y44 = -Y21;
    Y45 = 0;
    Y46 = Y33;
    Y47 = -Y24;
    Y48 = Y32;
    Y49 = -Y22;
    Y410 = -t5 + t6;
    Y411 = t17 - t13 + dwxr;
    Y412 = -t13;
    Y413 = t17;
    Y51 = 0;
    Y52 = -Y43;
    Y53 = 0;
    Y54 = Y11;
    Y55 = -Y48;
    Y56 = 0;
    Y57 = Y14;
    Y58 = -Y46;
    Y59 = t12 - t6;
    Y510 = Y13;
    Y511 = t8;
    Y512 = -t16 + Y511 + dwyr;
    Y513 = -t16;
    Y61 = 0;
    Y62 = Y21;
    Y63 = -Y54;
    Y64 = 0;
    Y65 = Y22;
    Y66 = -Y510;
    Y67 = 0;
    Y68 = -t12 + t5;
    Y69 = Y24;
    Y610 = -Y57;
    Y611 = -t7;
    Y612 = t11;
    Y613 = Y612 + Y611 + dwzr;
    
    
    YB41r = [Y11 Y12 Y13 Y14 Y15 Y16 Y17 Y18 Y19 Y110 Y111 Y112 Y113;...
             Y21 Y22 Y23 Y24 Y25 Y26 Y27 Y28 Y29 Y210 Y211 Y212 Y213;...
             Y31 Y32 Y33 Y34 Y35 Y36 Y37 Y38 Y39 Y310 Y311 Y312 Y313;...
             Y41 Y42 Y43 Y44 Y45 Y46 Y47 Y48 Y49 Y410 Y411 Y412 Y413;...
             Y51 Y52 Y53 Y54 Y55 Y56 Y57 Y58 Y59 Y510 Y511 Y512 Y513;...
             Y61 Y62 Y63 Y64 Y65 Y66 Y67 Y68 Y69 Y610 Y611 Y612 Y613];

end

== matlab function SimForces2022a/sbVDCController/sbAuxiliaryJointAngles/q2Angle ==
  data: theta2Filt input; q2 output; geom parameter
function q2 = q2Angle(theta2Filt, geom)

    % Calculates q2 angle value from the encoder- (or other by means-)
    % obtained angle Theta2.
    q2 = theta2Filt - geom.beta3 - geom.beta4;

end

== matlab function SimForces2022a/sbVDCController/sbFormTotalRequiredForces/sbTotalRequiredForcesRS1/regressorYBc1r ==
  data: Bc1V input; Bc1dV input; Bc1_Rot_W input; gravity parameter; YBc1r output
function YBc1r  = inertiaRegressor(Bc1V, Bc1dV, Bc1_Rot_W,  gravity)

    % Forms regressor matrix YBc1r as described in Appendix A of
    % Zhu, Wen-Hong. Virtual decomposition control: toward hyper degrees
    % of freedom robots. Vol. 60. Springer Science & Business Media, 2010.

    % The code below is not the most apparent 1-to-1 visual mapping to the
    % book equations since it was generated using a symbolic toolbox.

    vxr = Bc1V(1); vyr = Bc1V(2); vzr = Bc1V(3);
    wxr = Bc1V(4); wyr = Bc1V(5); wzr = Bc1V(6);
    
    axr = Bc1dV(1); ayr = Bc1dV(2); azr = Bc1dV(3);
    dwxr = Bc1dV(4); dwyr = Bc1dV(5); dwzr = Bc1dV(6);
    
    wx = Bc1V(4); wy = Bc1V(5); wz = Bc1V(6);
    
    Bc1g = Bc1_Rot_W*gravity.Wg;
    
    gx = Bc1g(1); gy = Bc1g(2); gz = Bc1g(3);
    
    Y11 = (-vyr * wz + vzr * wy + axr + gx);
    t5 = (wy * wyr);
    t6 = (wz * wzr);
    Y12 = -t5 - t6;
    t7 = (wxr * wy);
    Y13 = (t7 - dwzr);
    t8 = (wxr * wz);
    Y14  = (t8 + dwyr);
    Y15 = 0;
    Y16 = 0;
    Y17 = 0;
    Y18  = 0;
    Y19 = 0;
    Y110 = 0;
    Y111 = 0;
    Y112 = 0;
    Y113 = 0;
    Y21 = vxr * wz - vzr * wx + ayr + gy;
    t11 = wx * wyr;
    Y22 = t11 + dwzr;
    t12 = wx * wxr;
    Y23 = -t12 - t6;
    t13 = wyr * wz;
    Y24 = t13 - dwxr;
    Y25 = 0;
    Y26 = 0;
    Y27 = 0;
    Y28 = 0;
    Y29 = 0;
    Y210 = 0;
    Y211 = 0;
    Y212 = 0;
    Y213 = 0;
    Y31 = -vxr * wy + vyr * wx + azr + gz;
    t16 = wx * wzr;
    Y32 = t16 - dwyr;
    t17 = wy * wzr;
    Y33 = t17 + dwxr;
    Y34 = -t12 - t5;
    Y35 = 0;
    Y36 = 0;
    Y37 = 0;
    Y38 = 0;
    Y39 = 0;
    Y310 = 0;
    Y311 = 0;
    Y312 = 0;
    Y313 = 0;
    Y41 = 0;
    Y42 = 0;
    Y43 = Y31;
    Y44 = -Y21;
    Y45 = 0;
    Y46 = Y33;
    Y47 = -Y24;
    Y48 = Y32;
    Y49 = -Y22;
    Y410 = -t5 + t6;
    Y411 = t17 - t13 + dwxr;
    Y412 = -t13;
    Y413 = t17;
    Y51 = 0;
    Y52 = -Y43;
    Y53 = 0;
    Y54 = Y11;
    Y55 = -Y48;
    Y56 = 0;
    Y57 = Y14;
    Y58 = -Y46;
    Y59 = t12 - t6;
    Y510 = Y13;
    Y511 = t8;
    Y512 = -t16 + Y511 + dwyr;
    Y513 = -t16;
    Y61 = 0;
    Y62 = Y21;
    Y63 = -Y54;
    Y64 = 0;
    Y65 = Y22;
    Y66 = -Y510;
    Y67 = 0;
    Y68 = -t12 + t5;
    Y69 = Y24;
    Y610 = -Y57;
    Y611 = -t7;
    Y612 = t11;
    Y613 = Y612 + Y611 + dwzr;
    
    
    YBc1r = [Y11 Y12 Y13 Y14 Y15 Y16 Y17 Y18 Y19 Y110 Y111 Y112 Y113;...
             Y21 Y22 Y23 Y24 Y25 Y26 Y27 Y28 Y29 Y210 Y211 Y212 Y213;...
             Y31 Y32 Y33 Y34 Y35 Y36 Y37 Y38 Y39 Y310 Y311 Y312 Y313;...
             Y41 Y42 Y43 Y44 Y45 Y46 Y47 Y48 Y49 Y410 Y411 Y412 Y413;...
             Y51 Y52 Y53 Y54 Y55 Y56 Y57 Y58 Y59 Y510 Y511 Y512 Y513;...
             Y61 Y62 Y63 Y64 Y65 Y66 Y67 Y68 Y69 Y610 Y611 Y612 Y613];

end

== matlab function SimForces2022a/sbVDCController/sbFormAnalyticQuantities/sbRevoluteSegment1/sbGeomPropRS1/sbq12AngleValue/q12AngleValue ==
  data: x1 input; q12 output; geom parameter; cyl1 parameter
function q12 = q12AngleValue(x1, geom, cyl1)

    % Calculates q12-angle per the paper equation (20).
    q12 = -acos((geom.L1*geom.L1-(x1+cyl1.x0)*(x1+cyl1.x0)-geom.L11*geom.L11)/(-2*(x1+cyl1.x0)*geom.L11));

end

== matlab function SimForces2022a/sbVDCController/sbFormAnalyticQuantities/sbRevoluteSegment2/sbGeomPropRS2/sbq21AngleValue/q21AngleValue ==
  data: x2 input; q21 output; geom parameter; cyl2 parameter
function q21 = q21AngleValue(x2, geom, cyl2)

    % Calculates q21-angle per the paper equation (19).
    q21 = -acos((geom.L21*geom.L21-(x2+cyl2.x0)*(x2+cyl2.x0)-geom.L2*geom.L2)/(-2*(x2+cyl2.x0)*geom.L2));

end

== matlab function SimForces2022a/sbVDCController/sbFormAnalyticQuantities/sbRevoluteSegment2/sbGeomPropRS2/sbq21AngleRate/q21AngleRate ==
  data: x2 input; q21 input; dx2 input; dq21 output; geom parameter; cyl2 parameter
function dq21 = q21AngleRate(x2, q21, dx2, geom, cyl2)
    
    % Calculates q21 angle rate per the paper equation (22).
    dq21 = -((x2+cyl2.x0)-geom.L2*cos(q21))/((x2+cyl2.x0)*geom.L2*sin(q21))*dx2;

end

== matlab function SimForces2022a/sbVDCController/sbFormAnalyticQuantities/sbRevoluteSegment2/sbGeomPropRS2/sbTiltPistonVelocity/tiltPistonVelocity ==
  data: dq2 input; x2 input; q2 input; dx2 output; geom parameter; cyl2 parameter
function dx2 = tiltPistonVelocity(dq2, x2, q2, geom, cyl2)

    % Calculates lift piston velocity per the paper equation (21).
    dx2 = -(geom.L2*geom.L21*sin(q2))/(x2+cyl2.x0)*dq2;

end

== matlab function SimForces2022a/sbVDCController/sbFormAnalyticQuantities/sbRevoluteSegment2/sbGeomPropRS2/sbq22AngleValue/q22AngleValue ==
  data: x2 input; q22 output; geom parameter; cyl2 parameter
function q22 = q22AngleValue(x2, geom, cyl2)

    % Calculates q22-angle per the paper equation (20).
    q22 = -acos((geom.L2*geom.L2-(x2+cyl2.x0)*(x2+cyl2.x0)-geom.L21*geom.L21)/(-2*(x2+cyl2.x0)*geom.L21));

end
